simulink subsystem "BrakingHydraulics"  (R2025b)
settings: Solver=VariableStepAuto  StartTime=0.0  StopTime=10.0  RelTol=1e-3
undefined symbols (not defined in the file): PlntBrkFrntBias, PlntBrkPrsFctr, PlntBrkRearBias
libraries: autolibutils x1
settings Model: ModifiedByFormat=The MathWorks, Inc.  Creator=The MathWorks, Inc.  LastModifiedBy=The MathWorks, Inc.
settings OptimizationCC: ReuseModelBlockBuffer=off
settings RTWCC: GPUComputeCapability=3.5

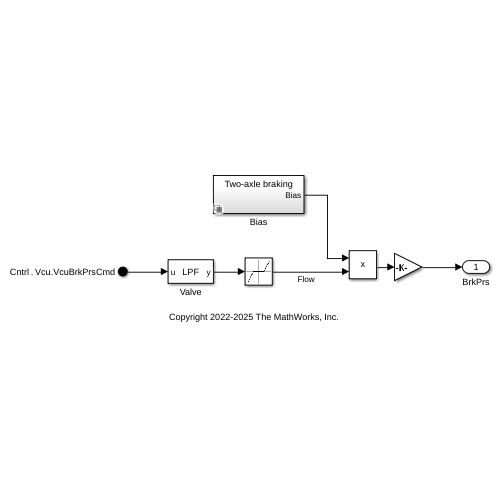
[thumbnail: Simulink's stored preview of the top-level diagram]
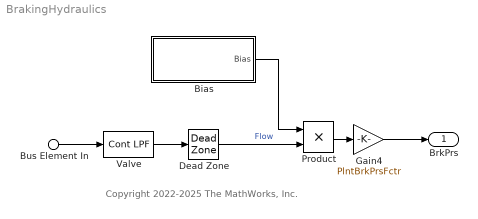
== system BrakingHydraulics ==
  note: Copyright 2022-2025 The MathWorks, Inc.
  Bus Element In : Inport  PortName=Cntrl  Element=Vcu.VcuBrkPrsCmd
  Bias : Subsystem  Variant=on  VariantControlMode=label  LabelModeActiveChoice=TwoAxleBraking
  Dead Zone : DeadZone  LowerValue=-inf  UpperValue=1e-3  ZeroCross=off
  Gain4 : Gain  Gain=PlntBrkPrsFctr
  Product : Product
  Valve : autolibutils/Cont LPF  wc=PlntBrkWc  AbsoluteTolerance=auto  aMode=6
  BrkPrs : Outport  VectorParamsAs1DForOutWhenUnconnected=off
  wires:
  Bias/1(Bias) -> Product/1
  Bus Element In/1 -> Valve/1
  Product/1 -> Gain4/1
  Valve/1 -> Dead Zone/1
  Gain4/1 -> BrkPrs/1
  Dead Zone/1 -> Product/2  "Flow"

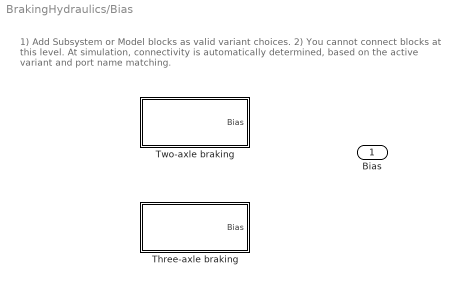
== system BrakingHydraulics/Bias ==
  note: 1) Add Subsystem or Model blocks as valid variant choices.
      | 2) You cannot connect blocks at this level. At simulation, connectivity is automatically
      | determined, based on the active variant and port name matching.
  Three-axle braking : Subsystem  VariantControl=ThreeAxleBraking
  Two-axle braking : Subsystem  VariantControl=TwoAxleBraking
  Bias : Outport

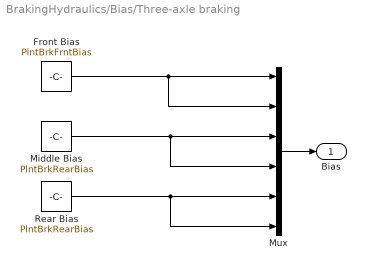
== system BrakingHydraulics/Bias/Three-axle braking ==
  Front Bias : Constant  Value=PlntBrkFrntBias  SampleTime=-1
  Middle Bias : Constant  Value=PlntBrkRearBias  SampleTime=-1
  Mux : Mux  Inputs=6
  Rear Bias : Constant  Value=PlntBrkRearBias  SampleTime=-1
  Bias : Outport
  wires:
  Rear Bias/1 -> Mux/6, Mux/5
  Front Bias/1 -> Mux/2, Mux/1
  Mux/1 -> Bias/1
  Middle Bias/1 -> Mux/4, Mux/3

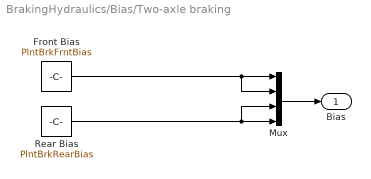
== system BrakingHydraulics/Bias/Two-axle braking ==
  Front Bias : Constant  Value=PlntBrkFrntBias  SampleTime=-1
  Mux : Mux
  Rear Bias : Constant  Value=PlntBrkRearBias  SampleTime=-1
  Bias : Outport
  wires:
  Rear Bias/1 -> Mux/3, Mux/4
  Front Bias/1 -> Mux/2, Mux/1
  Mux/1 -> Bias/1
